simulink model "ammclib_gflib_miscellaneous_s32k14x"  (Simulink 9.0)
settings: Solver=FixedStepDiscrete  StartTime=0.0  StopTime=10  FixedStep=0.001  RelTol=1e-3  EnableMultiTasking=on
InitFcn:
  | mbd_s32k_consistency_checks(bdroot(gcs));
undefined symbols (not defined in the file or in its folder): LQFP
libraries: ammclib_bam_s32k14x x27, simulink x7, mbd_s32k1xx_ec_toolbox x2
Description:
  | This model tests the AMMCLIB GFLIB SQRT, SIGN, HYST, RAMP and INTEGRATOR blocks
  | 
  | Validation:
  | - Run the model in Simulation and compare the Inputs vs Outputs results.
  | - Open Freemaster (ammclib_gflib_miscellaneous_s32k14x.pmp) and compare the HW results against the Simulated ones
settings Model: Creator=NXP MBDT Team  LastModifiedBy=nxf35172
settings DataIOCC: ExternalInput=off  InitialState=off  LimitDataPoints=on  SaveOutput=off  SignalLogging=off  SaveTime=off
settings OptimizationCC: DefaultParameterBehavior=Inlined  LifeSpan=1
settings DebuggingCC: SolverPrmCheckMsg=warning  InheritedTsInSrcMsg=none  SingleTaskRateTransMsg=error  ParameterPrecisionLossMsg=none  UnconnectedInputMsg=error  UnconnectedOutputMsg=error  UnconnectedLineMsg=error  AllowSymbolicDim=off  UnknownTsInhSupMsg=error  StateNameClashWarn=warning
settings HardwareCC: ProdLargestAtomicInteger=Long  ProdLargestAtomicFloat=Double  ProdEndianess=LittleEndian  ProdHWDeviceType=ARM Compatible->ARM Cortex
settings SFSimCC: MATLABDynamicMemAlloc=off
settings RTWCC: SystemTargetFile=mbd_s32k.tlc  MakeCommand=mbd_s32k_make_rtw COPY_MDLREF_INCLUDES=0  TemplateMakefile=mbd_s32k.tmf  Description=Model Based Design Toolbox S32K14x Code Generation Target
settings CodeAppCC: IgnoreCustomStorageClasses=off
settings STFCustomTargetCC: CombineOutputUpdateFcns=on  ERTCustomFileBanners=on  SupportContinuousTime=off  SupportNonInlinedSFcns=off  RemoveResetFunc=on  MATLABClassNameForMDSCustomization=Simulink.SoftwareTarget.ERTCustomization  GRTInterface=off  SystemTargetFile=mbd_s32k14.tlc
settings ERTTargetCC: MultiwordLength=2048  ParMdlRefBuildCompliant=off  CompOptLevelCompliant=off  ConcurrentExecutionCompliant=off  ModelStepFunctionPrototypeControlCompliant=off  CPPClassGenCompliant=off  UseToolchainInfoCompliant=off  InlinedParameterPlacement=NonHierarchical  ERTCustomFileTemplate=example_file_process.tlc  ConvertIfToSwitch=off  SuppressUnreachableDefaultCases=off

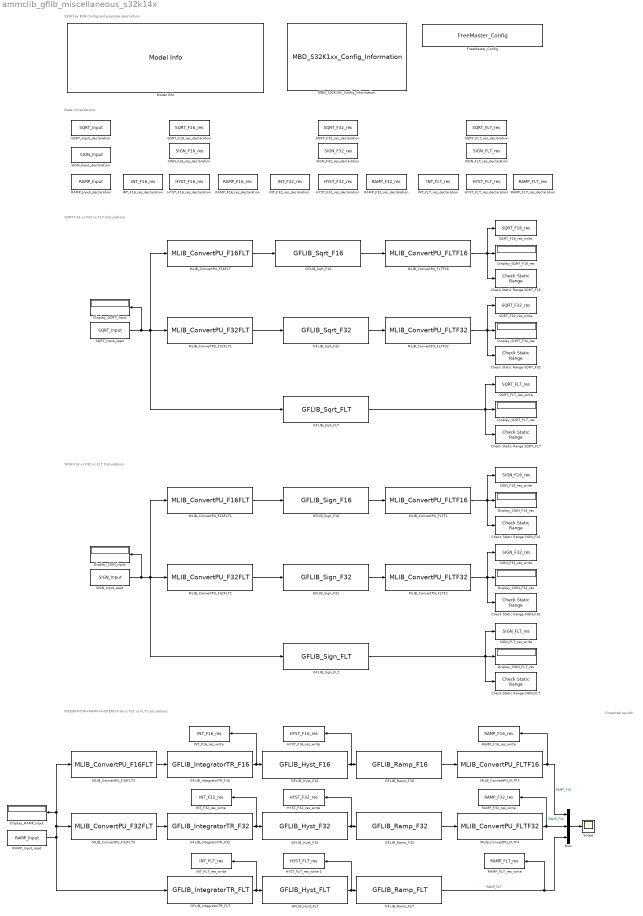
== system ammclib_gflib_miscellaneous_s32k14x ==
  note: Expected results:
  note: S32K14x EVB Config and example description
  note: Data Initializations
  note: SQRT F16 vs F32 vs FLT Calculations
  note: SIGN F16 vs F32 vs FLT Calculations
  note: INTEGRATOR+RAMP+HISTERIS F16 vs F32 vs FLT Calculations
  "Check Static Range SIGN_F16 " : simulink/Model Verification/Check  Static Range  Description=-1 <= u <= 1  max=1  max_included=on  min=-1  min_included=on  enabled=on  stopWhenAssertionFail=on  export=off  icon=graphic
      settings: SourceProductName=Simulink  SourceProductBaseCode=SL
  Check Static Range SIGN_F32 : simulink/Model Verification/Check  Static Range  Description=-1 <= u <= 1  max=1  max_included=on  min=-1  min_included=on  enabled=on  stopWhenAssertionFail=on  export=off  icon=graphic
      settings: SourceProductName=Simulink  SourceProductBaseCode=SL
  "Check Static Range SIGN_FLT  " : simulink/Model Verification/Check  Static Range  Description=-1 <= u <= 1  max=1  max_included=on  min=-1  min_included=on  enabled=on  stopWhenAssertionFail=on  export=off  icon=graphic
      settings: SourceProductName=Simulink  SourceProductBaseCode=SL
  "Check Static Range SQRT_F16 " : simulink/Model Verification/Check  Static Range  Description=0.7 <= u <= 0.8  max=0.8  max_included=on  min=0.7  min_included=on  enabled=on  stopWhenAssertionFail=on  export=off  icon=graphic
      settings: SourceProductName=Simulink  SourceProductBaseCode=SL
  Check Static Range SQRT_F32 : simulink/Model Verification/Check  Static Range  Description=0.7 <= u <= 0.8  max=0.8  max_included=on  min=0.7  min_included=on  enabled=on  stopWhenAssertionFail=on  export=off  icon=graphic
      settings: SourceProductName=Simulink  SourceProductBaseCode=SL
  Check Static Range SQRT_FLT : simulink/Model Verification/Check  Static Range  Description=0.7 <= u <= 0.8  max=0.8  max_included=on  min=0.7  min_included=on  enabled=on  stopWhenAssertionFail=on  export=off  icon=graphic
      settings: SourceProductName=Simulink  SourceProductBaseCode=SL
  Display_RAMP_input : Display
  Display_SIGN_F16_res : Display
  Display_SIGN_F32_res : Display
  Display_SIGN_FLT_res : Display
  Display_SIGN_input : Display
  Display_SQRT_F16_res : Display
  Display_SQRT_F32_res : Display
  Display_SQRT_FLT_res : Display
  Display_SQRT_input : Display
  FreeMaster_Config : mbd_s32k1xx_ec_toolbox/Utility Blocks/FreeMaster_Config  interface=LPUART1  baudrate=115200  rxd=PTC6: [LPUART1_RX | Receive]  txd=PTC7: [LPUART1_TX | Transmit]  mode=Short Interrupt  isr_prio=15  show_adv_opts=off  use_scope=on  max_scope_vars=8  use_recorder=on  max_rec_vars=8  rec_buff_size=1024  rec_timebase=0 milliseconds  comm_buffer_size_auto=on  comm_buffer_size=255  comm_rqueue_size_default=on  comm_rqueue_size=32
  GFLIB_Hyst_F16 : ammclib_bam_s32k14x/GFLIB/bam_f16/GFLIB_Hyst_F16  f16HystOn=(2^15-1)/2  f16HystOff=-(2^15-1)/2  f16OutValOn=0.03*(2^15-1)  f16OutValOff=-0.03*(2^15-1)
  GFLIB_Hyst_F32 : ammclib_bam_s32k14x/GFLIB/bam_f32/GFLIB_Hyst_F32  f32HystOn=(2^31-1)/2  f32HystOff=-(2^31-1)/2  f32OutValOn=0.03*(2^31-1)  f32OutValOff=-0.03*(2^31-1)
  GFLIB_Hyst_FLT : ammclib_bam_s32k14x/GFLIB/bam_flt/GFLIB_Hyst_FLT  fltHystOn=0.5  fltHystOff=-0.5  fltOutValOn=0.03  fltOutValOff=-0.03
  GFLIB_IntegratorTR_F16 : ammclib_bam_s32k14x/GFLIB/bam_f16/GFLIB_IntegratorTR_F16  f16C1=0.003*(2^15-1)  u16NShift=0
  GFLIB_IntegratorTR_F32 : ammclib_bam_s32k14x/GFLIB/bam_f32/GFLIB_IntegratorTR_F32  f32C1=0.003*(2^31-1)  u16NShift=0
  GFLIB_IntegratorTR_FLT : ammclib_bam_s32k14x/GFLIB/bam_flt/GFLIB_IntegratorTR_FLT  fltC1=0.003
  GFLIB_Ramp_F16 : ammclib_bam_s32k14x/GFLIB/bam_f16/GFLIB_Ramp_F16  f16RampUp=0.0001*(2^15-1)  f16RampDown=0.0001*(2^15-1)
  GFLIB_Ramp_F32 : ammclib_bam_s32k14x/GFLIB/bam_f32/GFLIB_Ramp_F32  f32RampUp=0.0001*(2^31-1)  f32RampDown=0.0001*(2^31-1)
  GFLIB_Ramp_FLT : ammclib_bam_s32k14x/GFLIB/bam_flt/GFLIB_Ramp_FLT  fltRampUp=0.0001  fltRampDown=0.0001
  GFLIB_Sign_F16 : ammclib_bam_s32k14x/GFLIB/bam_f16/GFLIB_Sign_F16
  GFLIB_Sign_F32 : ammclib_bam_s32k14x/GFLIB/bam_f32/GFLIB_Sign_F32
  GFLIB_Sign_FLT : ammclib_bam_s32k14x/GFLIB/bam_flt/GFLIB_Sign_FLT
  GFLIB_Sqrt_F16 : ammclib_bam_s32k14x/GFLIB/bam_f16/GFLIB_Sqrt_F16
  GFLIB_Sqrt_F32 : ammclib_bam_s32k14x/GFLIB/bam_f32/GFLIB_Sqrt_F32
  GFLIB_Sqrt_FLT : ammclib_bam_s32k14x/GFLIB/bam_flt/GFLIB_Sqrt_FLT
  HYST_F16_res_declaration : DataStoreMemory  Priority=2  DataStoreName=HYST_F16_res  ReadBeforeWriteMsg=warning  WriteAfterWriteMsg=warning  WriteAfterReadMsg=warning  ShowAdditionalParam=off  OutDataTypeStr=int16
  HYST_F16_res_write : DataStoreWrite  DataStoreName=HYST_F16_res
  HYST_F32_res_declaration : DataStoreMemory  Priority=2  DataStoreName=HYST_F32_res  ReadBeforeWriteMsg=warning  WriteAfterWriteMsg=warning  WriteAfterReadMsg=warning  ShowAdditionalParam=off  OutDataTypeStr=int32
  HYST_F32_res_write : DataStoreWrite  DataStoreName=HYST_F32_res
  "HYST_FLT_res_declaration " : DataStoreMemory  Priority=2  DataStoreName=HYST_FLT_res  ReadBeforeWriteMsg=warning  WriteAfterWriteMsg=warning  WriteAfterReadMsg=warning  ShowAdditionalParam=off  OutDataTypeStr=single
  HYST_FLT_res_write 1 : DataStoreWrite  DataStoreName=HYST_FLT_res
  INT_F16_res_declaration : DataStoreMemory  Priority=2  DataStoreName=INT_F16_res  ReadBeforeWriteMsg=warning  WriteAfterWriteMsg=warning  WriteAfterReadMsg=warning  ShowAdditionalParam=off  OutDataTypeStr=int16
  INT_F16_res_write : DataStoreWrite  DataStoreName=INT_F16_res
  INT_F32_res_declaration : DataStoreMemory  Priority=2  DataStoreName=INT_F32_res  ReadBeforeWriteMsg=warning  WriteAfterWriteMsg=warning  WriteAfterReadMsg=warning  ShowAdditionalParam=off  OutDataTypeStr=int32
  INT_F32_res_write : DataStoreWrite  DataStoreName=INT_F32_res
  "INT_FLT_res_declaration " : DataStoreMemory  Priority=2  DataStoreName=INT_FLT_res  ReadBeforeWriteMsg=warning  WriteAfterWriteMsg=warning  WriteAfterReadMsg=warning  ShowAdditionalParam=off  OutDataTypeStr=single
  "INT_FLT_res_write " : DataStoreWrite  DataStoreName=INT_FLT_res
  MBD_S32K14x_Config_Information : mbd_s32k1xx_ec_toolbox/MBD_S32K1xx_Config_Information  Priority=0  mbdt_ver=0  disp_str=|  config_params=[]  mcu_target_name=S32K144  mcu_target_package=100-LQFP  mcu_target_sram_size=64KB  mcu_system_clock_freq=80  mcu_xtal_freq=External 8  mcu_steptick_timer=LPIT Channel 0  mcu_steptick_prio=15  ds_import_enable=on  target_compiler=GCC  target_memory=FLASH  gcc_target_compile_opts=-mcpu=cortex-m4 -mthumb -mfloat-abi=hard -mfpu=fpv4-sp-d16 -O1 -g -gstrict-dwarf  gcc_target_assemble_opts=-mcpu=cortex-m4 -mthumb -mfloat-abi=hard -mfpu=fpv4-sp-d16 -g  gcc_target_link_opts=-mcpu=cortex-m4 -mthumb -mfloat-abi=hard -mfpu=fpv4-sp-d16  gcc_target_default_lcf=on  gcc_target_user_lcf=S32K144_64_flash.ld  ghs_target_compile_opts=-cpu=cortexm4f -thumb -DARM_MATH_CM4 -fpu=vfpv4_d16 -fsingle -Ogeneral -Wundef -Wimplicit-int -Wshadow -Wtrigraphs --no_commons --gnu_asm -gnu99 -gdwarf-2 -G  ghs_target_assemble_opts=-cpu=cortexm4f -fpu=vfpv4_d16  ghs_target_link_opts=-cpu=cortexm4f -thumb -fpu=vfpv4_d16  ghs_target_default_lcf=off  ghs_target_user_lcf=S32K144_64_flash.ld  iar_target_compile_opts=--cpu=Cortex-M4F --thumb --fpu=VFPv4_sp -Ol -e --debug --dlib_config normal  iar_target_assemble_opts=--cpu Cortex-M4F --thumb --fpu VFPv4_sp  iar_target_link_opts=--no_exceptions --vfe --inline  iar_target_default_lcf=off  iar_target_user_lcf=S32K144_64_flash.icf  pil_download_enable=off  rbl_download_enable=on  rbl_start_delay=5000000  rbl_download_interface=OpenSDA  rbl_restart_request=off  rbl_com_port=Custom  rbl_com_port_custom=COM1  pil_download_rate=57600  pil_opensda_drive=Custom  pil_opensda_drive_custom=D  pil_uart_instance=0  pil_uart_rx=PTA2: [LPUART0_RX | Receive]  pil_uart_tx=PTA3: [LPUART0_TX | Transmit]  FTM_PWM_PcrCheckEnDis=on  FTM_Input_Edge_Inputs_PcrCheckEnDis=on  FTM_Dual_Edge_Inputs_PcrCheckEnDis=on  FTM_Quadrature_Inputs_PcrCheckEnDis=on  FTM_Hall_Sensor_Inputs_PcrCheckEnDis=on  LPTMR_PcrCheckEnDis=on  PIT_PcrCheckEnDis=on  RTC_PcrCheckEnDis=on  FlexCAN_PcrCheckEnDis=on  LIN_PcrCheckEnDis=on  FlexIO_PcrCheckEnDis=on  LPI2C_PcrCheckEnDis=on  LPSPI_PcrCheckEnDis=on  LPUART_PcrCheckEnDis=on  CMP_PcrCheckEnDis=on  GPIO_OutputPcrCheckEnDis=on  GPIO_InputPcrCheckEnDis=on  SBC_PcrCheckEnDis=on  AMMCLIB_PcrCheckEnDis=on  FM_PcrCheckEnDis=on  Profile_PcrCheckEnDis=on  ConfigParams_PcrCheckEnDis=on  ModelRef_PcrCheckEnDis=on  PDB0_PcrCheckEnDis=on  CSEc_PcrCheckEnDis=on  eDMA_PcrCheckEnDis=on  ADC_PcrCheckEnDis=on  WDOG_PcrCheckEnDis=on
      | Target : S32K142-16KB_SRAM
      | Package : 100-pin
      | System clock : 80 MHz
      | XTAL clock : External 8 MHz
      | Compiler : GCC
      | Target Type : FLASH
      | Download Code after build : (OpenSDA: E)
      | Step Tick Interrupt Priority : 15
  MLIB_ConvertPU_F16FLT : ammclib_bam_s32k14x/MLIB/bam_f16/MLIB_ConvertPU_F16FLT
  MLIB_ConvertPU_F16FLT1 : ammclib_bam_s32k14x/MLIB/bam_f16/MLIB_ConvertPU_F16FLT
  MLIB_ConvertPU_F16FLT2 : ammclib_bam_s32k14x/MLIB/bam_f16/MLIB_ConvertPU_F16FLT
  MLIB_ConvertPU_F32FLT1 : ammclib_bam_s32k14x/MLIB/bam_f32/MLIB_ConvertPU_F32FLT
  MLIB_ConvertPU_F32FLT2 : ammclib_bam_s32k14x/MLIB/bam_f32/MLIB_ConvertPU_F32FLT
  MLIB_ConvertPU_F32FLT3 : ammclib_bam_s32k14x/MLIB/bam_f32/MLIB_ConvertPU_F32FLT
  MLIB_ConvertPU_FLTF1 : ammclib_bam_s32k14x/MLIB/bam_flt/MLIB_ConvertPU_FLTF16
  MLIB_ConvertPU_FLTF16 : ammclib_bam_s32k14x/MLIB/bam_flt/MLIB_ConvertPU_FLTF16
  MLIB_ConvertPU_FLTF2 : ammclib_bam_s32k14x/MLIB/bam_flt/MLIB_ConvertPU_FLTF32
  MLIB_ConvertPU_FLTF3 : ammclib_bam_s32k14x/MLIB/bam_flt/MLIB_ConvertPU_FLTF16
  MLIB_ConvertPU_FLTF32 : ammclib_bam_s32k14x/MLIB/bam_flt/MLIB_ConvertPU_FLTF32
  MLIB_ConvertPU_FLTF4 : ammclib_bam_s32k14x/MLIB/bam_flt/MLIB_ConvertPU_FLTF32
  Model Info : simulink/Model-Wide Utilities/Model Info  Frame=off  DisplayStringWithTags=|  HorizontalTextAlignment=Left  LeftAlignmentValue=0.02
      | Model Name: %<ModelName>
      | 
      | Description: %<Description>
  Mux : Mux  Inputs=3
  RAMP_F16_res_declaration : DataStoreMemory  Priority=2  DataStoreName=RAMP_F16_res  ReadBeforeWriteMsg=warning  WriteAfterWriteMsg=warning  WriteAfterReadMsg=warning  ShowAdditionalParam=off  OutDataTypeStr=single
  RAMP_F16_res_write : DataStoreWrite  DataStoreName=RAMP_F16_res
  RAMP_F32_res_declaration : DataStoreMemory  Priority=2  DataStoreName=RAMP_F32_res  ReadBeforeWriteMsg=warning  WriteAfterWriteMsg=warning  WriteAfterReadMsg=warning  ShowAdditionalParam=off  OutDataTypeStr=single
  "RAMP_F32_res_write " : DataStoreWrite  DataStoreName=RAMP_F32_res
  RAMP_FLT_res_declaration : DataStoreMemory  Priority=2  DataStoreName=RAMP_FLT_res  ReadBeforeWriteMsg=warning  WriteAfterWriteMsg=warning  WriteAfterReadMsg=warning  ShowAdditionalParam=off  OutDataTypeStr=single
  "RAMP_FLT_res_write " : DataStoreWrite  DataStoreName=RAMP_FLT_res
  RAMP_Input_declaration : DataStoreMemory  Priority=1  DataStoreName=RAMP_Input  WriteAfterWriteMsg=warning  WriteAfterReadMsg=warning  InitialValue=0.1  ShowAdditionalParam=off  OutMin=-1  OutMax=1  OutDataTypeStr=single
  RAMP_Input_read : DataStoreRead  DataStoreName=RAMP_Input
  SIGN_F16_res_declaration : DataStoreMemory  Priority=2  DataStoreName=SIGN_F16_res  ReadBeforeWriteMsg=warning  WriteAfterWriteMsg=warning  WriteAfterReadMsg=warning  ShowAdditionalParam=off  OutDataTypeStr=single
  SIGN_F16_res_write : DataStoreWrite  DataStoreName=SIGN_F16_res
  SIGN_F32_res_declaration : DataStoreMemory  Priority=2  DataStoreName=SIGN_F32_res  ReadBeforeWriteMsg=warning  WriteAfterWriteMsg=warning  WriteAfterReadMsg=warning  ShowAdditionalParam=off  OutDataTypeStr=single
  SIGN_F32_res_write : DataStoreWrite  DataStoreName=SIGN_F32_res
  SIGN_FLT_res_declaration : DataStoreMemory  Priority=2  DataStoreName=SIGN_FLT_res  ReadBeforeWriteMsg=warning  WriteAfterWriteMsg=warning  WriteAfterReadMsg=warning  ShowAdditionalParam=off  OutDataTypeStr=single
  SIGN_FLT_res_write : DataStoreWrite  DataStoreName=SIGN_FLT_res
  SIGN_Input_declaration : DataStoreMemory  Priority=1  DataStoreName=SIGN_Input  WriteAfterWriteMsg=warning  WriteAfterReadMsg=warning  InitialValue=-0.5  ShowAdditionalParam=off  OutMin=-1  OutMax=1  OutDataTypeStr=single
  SIGN_Input_read : DataStoreRead  DataStoreName=SIGN_Input
  SQRT_F16_res_declaration : DataStoreMemory  Priority=2  DataStoreName=SQRT_F16_res  ReadBeforeWriteMsg=warning  WriteAfterWriteMsg=warning  WriteAfterReadMsg=warning  ShowAdditionalParam=off  OutDataTypeStr=single
  SQRT_F16_res_write : DataStoreWrite  DataStoreName=SQRT_F16_res
  SQRT_F32_res_declaration : DataStoreMemory  Priority=2  DataStoreName=SQRT_F32_res  ReadBeforeWriteMsg=warning  WriteAfterWriteMsg=warning  WriteAfterReadMsg=warning  ShowAdditionalParam=off  OutDataTypeStr=single
  SQRT_F32_res_write : DataStoreWrite  DataStoreName=SQRT_F32_res
  SQRT_FLT_res_declaration : DataStoreMemory  Priority=2  DataStoreName=SQRT_FLT_res  ReadBeforeWriteMsg=warning  WriteAfterWriteMsg=warning  WriteAfterReadMsg=warning  ShowAdditionalParam=off  OutDataTypeStr=single
  SQRT_FLT_res_write : DataStoreWrite  DataStoreName=SQRT_FLT_res
  SQRT_Input_declaration : DataStoreMemory  Priority=1  DataStoreName=SQRT_Input  WriteAfterWriteMsg=warning  WriteAfterReadMsg=warning  InitialValue=0.5  ShowAdditionalParam=off  OutMin=0  OutMax=1  OutDataTypeStr=single
  SQRT_Input_read : DataStoreRead  DataStoreName=SQRT_Input
  Scope : Scope
  wires:
  SQRT_Input_read/1 -> GFLIB_Sqrt_FLT/1, MLIB_ConvertPU_F32FLT1/1, MLIB_ConvertPU_F16FLT/1, Display_SQRT_input/1
  MLIB_ConvertPU_F16FLT/1 -> GFLIB_Sqrt_F16/1
  MLIB_ConvertPU_FLTF16/1 -> SQRT_F16_res_write/1, Display_SQRT_F16_res/1, "Check Static Range SQRT_F16 "/1
  GFLIB_Sqrt_F16/1 -> MLIB_ConvertPU_FLTF16/1
  MLIB_ConvertPU_F32FLT1/1 -> GFLIB_Sqrt_F32/1
  GFLIB_Sqrt_F32/1 -> MLIB_ConvertPU_FLTF32/1
  MLIB_ConvertPU_FLTF32/1 -> Check Static Range SQRT_F32/1, Display_SQRT_F32_res/1, SQRT_F32_res_write/1
  GFLIB_Sqrt_FLT/1 -> Check Static Range SQRT_FLT/1, Display_SQRT_FLT_res/1, SQRT_FLT_res_write/1
  SIGN_Input_read/1 -> GFLIB_Sign_FLT/1, MLIB_ConvertPU_F32FLT2/1, MLIB_ConvertPU_F16FLT1/1, Display_SIGN_input/1
  MLIB_ConvertPU_F16FLT1/1 -> GFLIB_Sign_F16/1
  MLIB_ConvertPU_FLTF1/1 -> SIGN_F16_res_write/1, Display_SIGN_F16_res/1, "Check Static Range SIGN_F16 "/1
  GFLIB_Sign_F16/1 -> MLIB_ConvertPU_FLTF1/1
  MLIB_ConvertPU_F32FLT2/1 -> GFLIB_Sign_F32/1
  GFLIB_Sign_F32/1 -> MLIB_ConvertPU_FLTF2/1
  MLIB_ConvertPU_FLTF2/1 -> Check Static Range SIGN_F32/1, Display_SIGN_F32_res/1, SIGN_F32_res_write/1
  GFLIB_Sign_FLT/1 -> "Check Static Range SIGN_FLT  "/1, Display_SIGN_FLT_res/1, SIGN_FLT_res_write/1
  RAMP_Input_read/1 -> MLIB_ConvertPU_F16FLT2/1, Display_RAMP_input/1, MLIB_ConvertPU_F32FLT3/1, GFLIB_IntegratorTR_FLT/1
  MLIB_ConvertPU_F16FLT2/1 -> GFLIB_IntegratorTR_F16/1
  GFLIB_IntegratorTR_F16/1 -> INT_F16_res_write/1, GFLIB_Hyst_F16/1
  GFLIB_Hyst_F16/1 -> HYST_F16_res_write/1, GFLIB_Ramp_F16/1
  GFLIB_Ramp_F16/1 -> MLIB_ConvertPU_FLTF3/1
  MLIB_ConvertPU_FLTF3/1 -> Mux/1, RAMP_F16_res_write/1  "RAMP_F16"
  MLIB_ConvertPU_F32FLT3/1 -> GFLIB_IntegratorTR_F32/1
  GFLIB_IntegratorTR_F32/1 -> INT_F32_res_write/1, GFLIB_Hyst_F32/1
  GFLIB_Hyst_F32/1 -> HYST_F32_res_write/1, GFLIB_Ramp_F32/1
  GFLIB_Ramp_F32/1 -> MLIB_ConvertPU_FLTF4/1
  MLIB_ConvertPU_FLTF4/1 -> Mux/2, "RAMP_F32_res_write "/1  "RAMP_F32"
  GFLIB_IntegratorTR_FLT/1 -> "INT_FLT_res_write "/1, GFLIB_Hyst_FLT/1
  GFLIB_Hyst_FLT/1 -> HYST_FLT_res_write 1/1, GFLIB_Ramp_FLT/1
  GFLIB_Ramp_FLT/1 -> "RAMP_FLT_res_write "/1, Mux/3  "RAMP_FLT"
  Mux/1 -> Scope/1
